simulink model "test_PF70mm"  (R2018b)
settings: Solver=FixedStepAuto  StartTime=0.0  StopTime=10  FixedStep=dt  RelTol=1e-3
undefined symbols (not defined in the file): dt
settings Model: Creator=39926  LastModifiedBy=39926

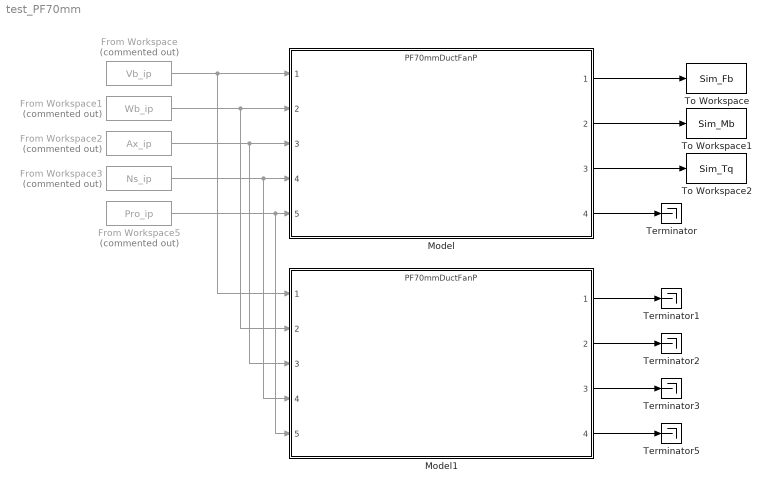
== system test_PF70mm ==
  From Workspace : FromWorkspace  Commented=on  VariableName=Vb_ip  SampleTime=dt
  From Workspace1 : FromWorkspace  Commented=on  VariableName=Wb_ip  SampleTime=dt
  From Workspace2 : FromWorkspace  Commented=on  VariableName=Ax_ip  SampleTime=dt
  From Workspace3 : FromWorkspace  Commented=on  VariableName=Ns_ip  SampleTime=dt
  From Workspace5 : FromWorkspace  Commented=on  VariableName=Pro_ip  SampleTime=dt
  Model : ModelReference  ModelNameDialog=PF70mmDuctFanP.slx  SimulationMode=Normal  ModelReferenceVersion=1.37
  Model1 : ModelReference  ModelNameDialog=PF70mmDuctFanP.slx  SimulationMode=Normal  ModelReferenceVersion=1.37
  Terminator{,1..3,5} (5 alike) : Terminator
  To Workspace : ToWorkspace  VariableName=Sim_Fb  SaveFormat=Timeseries  SampleTime=-1
  To Workspace1 : ToWorkspace  VariableName=Sim_Mb  SaveFormat=Timeseries  SampleTime=-1
  To Workspace2 : ToWorkspace  VariableName=Sim_Tq  SaveFormat=Timeseries  SampleTime=-1
  wires:
  From Workspace/1 -> Model/1, Model1/1
  From Workspace1/1 -> Model1/2, Model/2
  From Workspace2/1 -> Model1/3, Model/3
  From Workspace5/1 -> Model1/5, Model/5
  Model/1 -> To Workspace/1
  Model/2 -> To Workspace1/1
  Model/3 -> To Workspace2/1
  Model/4 -> Terminator/1
  From Workspace3/1 -> Model1/4, Model/4
  Model1/1 -> Terminator1/1
  Model1/2 -> Terminator2/1
  Model1/3 -> Terminator3/1
  Model1/4 -> Terminator5/1
